simulink model "SPWM"  (R2018a)
settings: Solver=FixedStepDiscrete  StartTime=0.0  StopTime=Inf  FixedStep=1e-5  RelTol=1e-3  EnableMultiTasking=on
undefined symbols (not defined in the file or in its folder): Down, GPTRIP1SEL, GPTRIP2SEL, TZ1, TZ2, Up
libraries: idelinklib_common x48, c2837xDlib x27, c2802xlib x2, c2000lib x1, simulink x1
(part 1 of 2)
settings Model: ExtModeTrigDuration=8  Creator=ThinkPad  LastModifiedBy=ThinkPad
settings OptimizationCC: DefaultUnderspecifiedDataType=single  EnhancedBackFolding=on  PassReuseOutputArgsAs=Individual arguments  MaxStackSize=512  OptimizeBlockOrder=speed  DifferentSizesBufferReuse=on  OptimizationCustomize=off
settings DebuggingCC: ParameterTunabilityLossMsg=error
settings HardwareCC: ProdBitPerChar=16  ProdBitPerInt=16  ProdBitPerPointer=32  ProdBitPerSizeT=32  ProdBitPerPtrDiffT=32  ProdLargestAtomicInteger=Integer  ProdLargestAtomicFloat=None  ProdWordSize=16  ProdLongLongMode=on  ProdHWDeviceType=Texas Instruments->C2000
settings SFSimCC: MATLABDynamicMemAlloc=off
settings RTWCC: SystemTargetFile=ert.tlc  HardwareBoard=TI Delfino F2837xD  TLCOptions=-aInlineSetEventsForThisBaseRateFcn=TLC_FALSE -aSuppressMultiTaskScheduler=TLC_FALSE -aRateBasedStepFcn=1  TemplateMakefile=ert_default_tmf  GenerateReport=on  Toolchain=Texas Instruments Code Composer Studio (C2000)  IncludeHyperlinkInReport=on  LaunchReport=on  GenerateTraceInfo=on  GenerateTraceReport=on  GenerateTraceReportSl=on  GenerateTraceReportSf=on  GenerateTraceReportEml=on
settings RTWCC: CustomHeaderCode=|
  | nt i=0;
  | #define AD_ADDRESS1 (int16 * )0x0081F00
settings CodeAppCC: ForceParamTrailComments=on  IgnoreCustomStorageClasses=off  OperatorAnnotations=on  SimulinkDataObjDesc=on  SFDataObjDesc=on  InsertBlockDesc=on
settings ERTTargetCC: TargetLangStandard=C99 (ISO)  CodeReplacementLibrary=TI C28x  RootIOFormat=Structure reference  EnableSignedLeftShifts=off

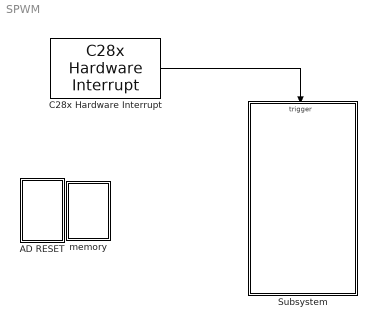
== system SPWM ==
  AD RESET : Subsystem
  C28x Hardware Interrupt : c2000lib/Scheduling/C28x Hardware Interrupt  irqnumbers=[3 1]  pienumbers=[1 2]  irqpriorities=[30 26]  irqpreempts=[0 0]  showinput=off  dspchiptype=C280X
      settings: SourceProductName=Embedded Coder Support Package for Texas Instruments C2000 Processors  SourceProductBaseCode=TIC2000
  Subsystem : Subsystem
  memory : Subsystem
  wires:
  C28x Hardware Interrupt/1 -> Subsystem/Trigger

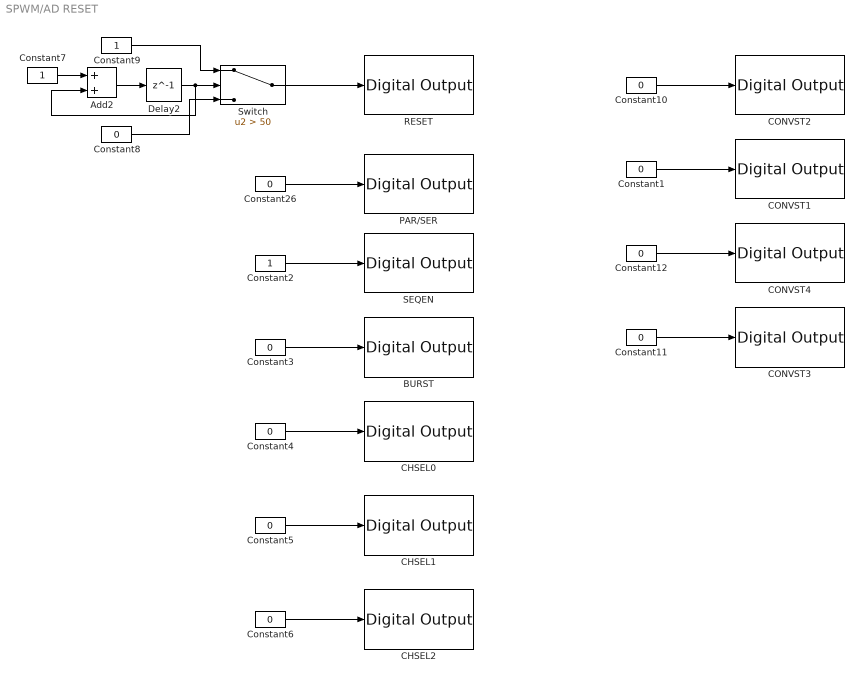
== system SPWM/AD RESET ==
  Add2 : Sum
  BURST : c2837xDlib/Digital Output  GPIO_Number=GPIO72~GPIO79  GPIO_Bit0=off  GPIO_BIT0_Toggle=off  GPIO_Bit1=off  GPIO_BIT1_Toggle=off  GPIO_Bit2=off  GPIO_BIT2_Toggle=off  GPIO_Bit3=off  GPIO_BIT3_Toggle=off  GPIO_Bit4=on  GPIO_BIT4_Toggle=off  GPIO_Bit5=off  GPIO_BIT5_Toggle=off  GPIO_Bit6=off  GPIO_BIT6_Toggle=off  GPIO_Bit7=off  GPIO_BIT7_Toggle=off
      settings: SourceProductName=Embedded Coder Support Package for Texas Instruments C2000 Processors  SourceProductBaseCode=TIC2000
  CHSEL0 : c2837xDlib/Digital Output  GPIO_Number=GPIO80~GPIO87  GPIO_Bit0=off  GPIO_BIT0_Toggle=off  GPIO_Bit1=off  GPIO_BIT1_Toggle=off  GPIO_Bit2=off  GPIO_BIT2_Toggle=off  GPIO_Bit3=on  GPIO_BIT3_Toggle=off  GPIO_Bit4=off  GPIO_BIT4_Toggle=off  GPIO_Bit5=off  GPIO_BIT5_Toggle=off  GPIO_Bit6=off  GPIO_BIT6_Toggle=off  GPIO_Bit7=off  GPIO_BIT7_Toggle=off
      settings: SourceProductName=Embedded Coder Support Package for Texas Instruments C2000 Processors  SourceProductBaseCode=TIC2000
  CHSEL1 : c2837xDlib/Digital Output  GPIO_Number=GPIO80~GPIO87  GPIO_Bit0=off  GPIO_BIT0_Toggle=off  GPIO_Bit1=on  GPIO_BIT1_Toggle=off  GPIO_Bit2=off  GPIO_BIT2_Toggle=off  GPIO_Bit3=off  GPIO_BIT3_Toggle=off  GPIO_Bit4=off  GPIO_BIT4_Toggle=off  GPIO_Bit5=off  GPIO_BIT5_Toggle=off  GPIO_Bit6=off  GPIO_BIT6_Toggle=off  GPIO_Bit7=off  GPIO_BIT7_Toggle=off
      settings: SourceProductName=Embedded Coder Support Package for Texas Instruments C2000 Processors  SourceProductBaseCode=TIC2000
  CHSEL2 : c2837xDlib/Digital Output  GPIO_Number=GPIO72~GPIO79  GPIO_Bit0=off  GPIO_BIT0_Toggle=off  GPIO_Bit1=off  GPIO_BIT1_Toggle=off  GPIO_Bit2=off  GPIO_BIT2_Toggle=off  GPIO_Bit3=off  GPIO_BIT3_Toggle=off  GPIO_Bit4=off  GPIO_BIT4_Toggle=off  GPIO_Bit5=off  GPIO_BIT5_Toggle=off  GPIO_Bit6=off  GPIO_BIT6_Toggle=off  GPIO_Bit7=on  GPIO_BIT7_Toggle=off
      settings: SourceProductName=Embedded Coder Support Package for Texas Instruments C2000 Processors  SourceProductBaseCode=TIC2000
  CONVST{1..4} (4 alike) : c2837xDlib/Digital Output  GPIO_Number=GPIO88~GPIO95  GPIO_Bit0=off  GPIO_BIT0_Toggle=off  GPIO_Bit1=on  GPIO_BIT1_Toggle=off  GPIO_Bit2=off  GPIO_BIT2_Toggle=off  GPIO_Bit3=off  GPIO_BIT3_Toggle=off  GPIO_Bit4=off  GPIO_BIT4_Toggle=off  GPIO_Bit5=off  GPIO_BIT5_Toggle=off  GPIO_Bit6=off  GPIO_BIT6_Toggle=off  GPIO_Bit7=off  GPIO_BIT7_Toggle=off
      settings: SourceProductName=Embedded Coder Support Package for Texas Instruments C2000 Processors  SourceProductBaseCode=TIC2000
  Constant{1,3..6,8,10..12,26} (10 alike) : Constant  Value=0  OutDataTypeStr=boolean
  Constant2 : Constant  OutDataTypeStr=boolean
  Constant7 : Constant  OutDataTypeStr=boolean
  Constant9 : Constant  OutDataTypeStr=boolean
  Delay2 : Delay  DelayLength=1
  PAR/SER : c2837xDlib/Digital Output  GPIO_Number=GPIO72~GPIO79  GPIO_Bit0=off  GPIO_BIT0_Toggle=off  GPIO_Bit1=off  GPIO_BIT1_Toggle=off  GPIO_Bit2=off  GPIO_BIT2_Toggle=off  GPIO_Bit3=off  GPIO_BIT3_Toggle=off  GPIO_Bit4=off  GPIO_BIT4_Toggle=off  GPIO_Bit5=off  GPIO_BIT5_Toggle=off  GPIO_Bit6=on  GPIO_BIT6_Toggle=off  GPIO_Bit7=off  GPIO_BIT7_Toggle=off
      settings: SourceProductName=Embedded Coder Support Package for Texas Instruments C2000 Processors  SourceProductBaseCode=TIC2000
  RESET : c2837xDlib/Digital Output  GPIO_Number=GPIO88~GPIO95  GPIO_Bit0=off  GPIO_BIT0_Toggle=off  GPIO_Bit1=off  GPIO_BIT1_Toggle=off  GPIO_Bit2=off  GPIO_BIT2_Toggle=off  GPIO_Bit3=off  GPIO_BIT3_Toggle=off  GPIO_Bit4=off  GPIO_BIT4_Toggle=off  GPIO_Bit5=on  GPIO_BIT5_Toggle=off  GPIO_Bit6=off  GPIO_BIT6_Toggle=off  GPIO_Bit7=off  GPIO_BIT7_Toggle=off
      settings: SourceProductName=Embedded Coder Support Package for Texas Instruments C2000 Processors  SourceProductBaseCode=TIC2000
  SEQEN : c2837xDlib/Digital Output  GPIO_Number=GPIO80~GPIO87  GPIO_Bit0=on  GPIO_BIT0_Toggle=off  GPIO_Bit1=off  GPIO_BIT1_Toggle=off  GPIO_Bit2=off  GPIO_BIT2_Toggle=off  GPIO_Bit3=off  GPIO_BIT3_Toggle=off  GPIO_Bit4=off  GPIO_BIT4_Toggle=off  GPIO_Bit5=off  GPIO_BIT5_Toggle=off  GPIO_Bit6=off  GPIO_BIT6_Toggle=off  GPIO_Bit7=off  GPIO_BIT7_Toggle=off
      settings: SourceProductName=Embedded Coder Support Package for Texas Instruments C2000 Processors  SourceProductBaseCode=TIC2000
  Switch : Switch  Criteria=u2 > Threshold  Threshold=50
  wires:
  Constant4/1 -> CHSEL0/1
  Delay2/1 -> Add2/2, Switch/2
  Constant5/1 -> CHSEL1/1
  Constant3/1 -> BURST/1
  Constant8/1 -> Switch/3
  Add2/1 -> Delay2/1
  Switch/1 -> RESET/1
  Constant7/1 -> Add2/1
  Constant6/1 -> CHSEL2/1
  Constant2/1 -> SEQEN/1
  Constant9/1 -> Switch/1
  Constant26/1 -> PAR/SER/1
  Constant10/1 -> CONVST2/1
  Constant1/1 -> CONVST1/1
  Constant11/1 -> CONVST3/1
  Constant12/1 -> CONVST4/1

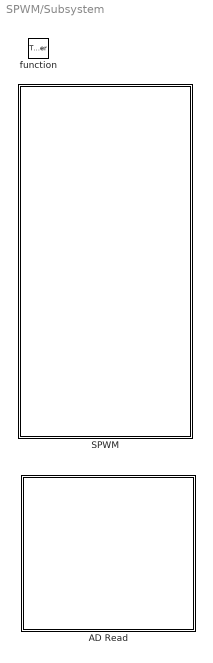
== system SPWM/Subsystem ==
  function : TriggerPort  TriggerType=function-call  VariantControl=(inherit)  SampleTime=1e-5
  AD Read : Subsystem
  SPWM : Subsystem

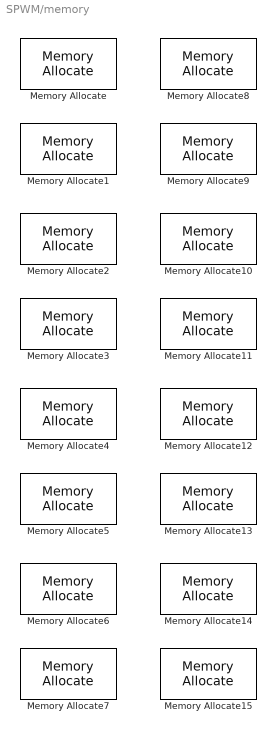
== system SPWM/memory ==
  Memory Allocate : idelinklib_common/Memory Allocate  variableName=V0A  alignThisVariable=off  memoryAlignmentBoundary=4  dataType=int16  specifyQualifier=off  typeQualifier=volatile  dataDimension=1  specifyMemorySection=off  memorySection=Sector A  bindMemorySection=on  sectionStartAddress=hex2dec('00080000')  initializeMemory=on  initialValue=0
  Memory Allocate1 : idelinklib_common/Memory Allocate  variableName=V0B  alignThisVariable=off  memoryAlignmentBoundary=4  dataType=int16  specifyQualifier=off  typeQualifier=volatile  dataDimension=1  specifyMemorySection=off  memorySection=Sector A  bindMemorySection=on  sectionStartAddress=hex2dec('00080000')  initializeMemory=on  initialValue=0
  Memory Allocate10 : idelinklib_common/Memory Allocate  variableName=V5A  alignThisVariable=off  memoryAlignmentBoundary=4  dataType=int16  specifyQualifier=off  typeQualifier=volatile  dataDimension=1  specifyMemorySection=off  memorySection=Sector A  bindMemorySection=on  sectionStartAddress=hex2dec('00080000')  initializeMemory=on  initialValue=0
  Memory Allocate11 : idelinklib_common/Memory Allocate  variableName=V5B  alignThisVariable=off  memoryAlignmentBoundary=4  dataType=int16  specifyQualifier=off  typeQualifier=volatile  dataDimension=1  specifyMemorySection=off  memorySection=Sector A  bindMemorySection=on  sectionStartAddress=hex2dec('00080000')  initializeMemory=on  initialValue=0
  Memory Allocate12 : idelinklib_common/Memory Allocate  variableName=V6A  alignThisVariable=off  memoryAlignmentBoundary=4  dataType=int16  specifyQualifier=off  typeQualifier=volatile  dataDimension=1  specifyMemorySection=off  memorySection=Sector A  bindMemorySection=on  sectionStartAddress=hex2dec('00080000')  initializeMemory=on  initialValue=0
  Memory Allocate13 : idelinklib_common/Memory Allocate  variableName=V6B  alignThisVariable=off  memoryAlignmentBoundary=4  dataType=int16  specifyQualifier=off  typeQualifier=volatile  dataDimension=1  specifyMemorySection=off  memorySection=Sector A  bindMemorySection=on  sectionStartAddress=hex2dec('00080000')  initializeMemory=on  initialValue=0
  Memory Allocate14 : idelinklib_common/Memory Allocate  variableName=V7A  alignThisVariable=off  memoryAlignmentBoundary=4  dataType=int16  specifyQualifier=off  typeQualifier=volatile  dataDimension=1  specifyMemorySection=off  memorySection=Sector A  bindMemorySection=on  sectionStartAddress=hex2dec('00080000')  initializeMemory=on  initialValue=0
  Memory Allocate15 : idelinklib_common/Memory Allocate  variableName=V7B  alignThisVariable=off  memoryAlignmentBoundary=4  dataType=int16  specifyQualifier=off  typeQualifier=volatile  dataDimension=1  specifyMemorySection=off  memorySection=Sector A  bindMemorySection=on  sectionStartAddress=hex2dec('00080000')  initializeMemory=on  initialValue=0
  Memory Allocate2 : idelinklib_common/Memory Allocate  variableName=V1A  alignThisVariable=off  memoryAlignmentBoundary=4  dataType=int16  specifyQualifier=off  typeQualifier=volatile  dataDimension=1  specifyMemorySection=off  memorySection=Sector A  bindMemorySection=on  sectionStartAddress=hex2dec('00080000')  initializeMemory=on  initialValue=0
  Memory Allocate3 : idelinklib_common/Memory Allocate  variableName=V1B  alignThisVariable=off  memoryAlignmentBoundary=4  dataType=int16  specifyQualifier=off  typeQualifier=volatile  dataDimension=1  specifyMemorySection=off  memorySection=Sector A  bindMemorySection=on  sectionStartAddress=hex2dec('00080000')  initializeMemory=on  initialValue=0
  Memory Allocate4 : idelinklib_common/Memory Allocate  variableName=V2A  alignThisVariable=off  memoryAlignmentBoundary=4  dataType=int16  specifyQualifier=off  typeQualifier=volatile  dataDimension=1  specifyMemorySection=off  memorySection=Sector A  bindMemorySection=on  sectionStartAddress=hex2dec('00080000')  initializeMemory=on  initialValue=0
  Memory Allocate5 : idelinklib_common/Memory Allocate  variableName=V2B  alignThisVariable=off  memoryAlignmentBoundary=4  dataType=int16  specifyQualifier=off  typeQualifier=volatile  dataDimension=1  specifyMemorySection=off  memorySection=Sector A  bindMemorySection=on  sectionStartAddress=hex2dec('00080000')  initializeMemory=on  initialValue=0
  Memory Allocate6 : idelinklib_common/Memory Allocate  variableName=V3A  alignThisVariable=off  memoryAlignmentBoundary=4  dataType=int16  specifyQualifier=off  typeQualifier=volatile  dataDimension=1  specifyMemorySection=off  memorySection=Sector A  bindMemorySection=on  sectionStartAddress=hex2dec('00080000')  initializeMemory=on  initialValue=0
  Memory Allocate7 : idelinklib_common/Memory Allocate  variableName=V3B  alignThisVariable=off  memoryAlignmentBoundary=4  dataType=int16  specifyQualifier=off  typeQualifier=volatile  dataDimension=1  specifyMemorySection=off  memorySection=Sector A  bindMemorySection=on  sectionStartAddress=hex2dec('00080000')  initializeMemory=on  initialValue=0
  Memory Allocate8 : idelinklib_common/Memory Allocate  variableName=V4A  alignThisVariable=off  memoryAlignmentBoundary=4  dataType=int16  specifyQualifier=off  typeQualifier=volatile  dataDimension=1  specifyMemorySection=off  memorySection=Sector A  bindMemorySection=on  sectionStartAddress=hex2dec('00080000')  initializeMemory=on  initialValue=0
  Memory Allocate9 : idelinklib_common/Memory Allocate  variableName=V4B  alignThisVariable=off  memoryAlignmentBoundary=4  dataType=int16  specifyQualifier=off  typeQualifier=volatile  dataDimension=1  specifyMemorySection=off  memorySection=Sector A  bindMemorySection=on  sectionStartAddress=hex2dec('00080000')  initializeMemory=on  initialValue=0

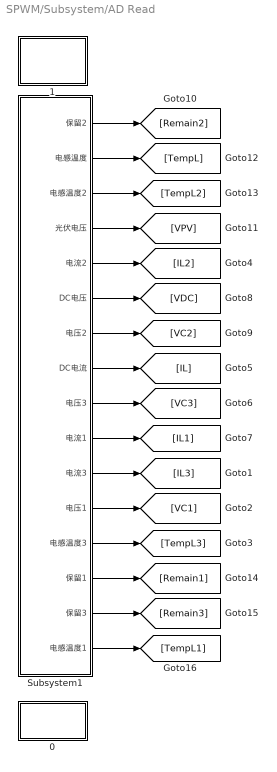
== system SPWM/Subsystem/AD Read ==
  0 : Subsystem
  1 : Subsystem
  Subsystem1 : Subsystem
  wires:
  Subsystem1/16(电感温度1) -> [TempL1]
  Subsystem1/15(保留3) -> [Remain3]
  Subsystem1/14(保留1) -> [Remain1]
  Subsystem1/13(电感温度3) -> [TempL3]
  Subsystem1/12(电压1) -> [VC1]
  Subsystem1/11(电流3) -> [IL3]
  Subsystem1/10(电流1) -> [IL1]
  Subsystem1/9(电压3) -> [VC3]
  Subsystem1/7(电压2) -> [VC2]
  Subsystem1/6(DC电压) -> [VDC]
  Subsystem1/5(电流2) -> [IL2]
  Subsystem1/3(电感温度2) -> [TempL2]
  Subsystem1/8(DC电流) -> [IL]
  Subsystem1/2(电感温度) -> [TempL]
  Subsystem1/4(光伏电压) -> [VPV]
  Subsystem1/1(保留2) -> [Remain2]

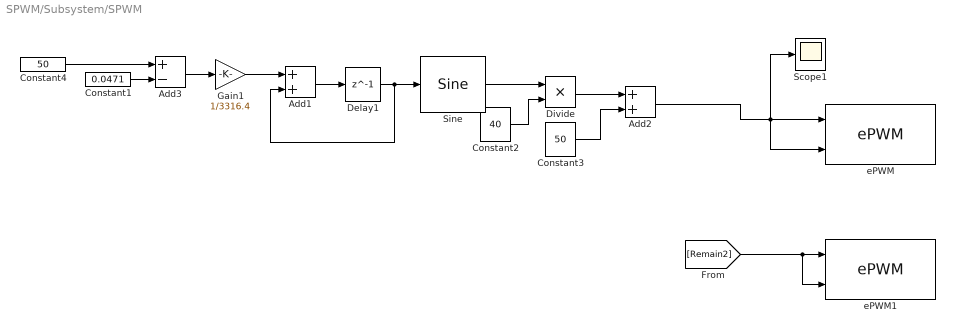
== system SPWM/Subsystem/SPWM ==
  Add1 : Sum
  Add2 : Sum
  Add3 : Sum  Inputs=+-
  Constant1 : Constant  Value=0.0471  VectorParams1D=off
  Constant2 : Constant  Value=40  VectorParams1D=off
  Constant3 : Constant  Value=50  VectorParams1D=off
  Constant4 : Constant  Value=50  VectorParams1D=off
  Delay1 : Delay  DelayLength=1
  Divide : Product  Inputs=**
  Gain1 : Gain  Gain=1/3316.4
  Scope1 : Scope
  Sine : simulink/Lookup Tables/Sine  Formula=sin(2*pi*u)  NumDataPoints=(2^5)+1  OutputWordLength=16  InternalRulePriority=Precision
      settings: SourceProductName=Simulink
  ePWM : c2802xlib/ePWM  useModule=ePWM1  ePWMxLINKTBPRD=Not Linked  periodUnits=Clock cycles  timerSource=Specify via dialog  timerPeriod_clk=15000  timerPeriod_sec=0.0001  tbshadow=Counter equals to zero  countingMode=Up-Down  phaseActiveEnable=Disable  phaseDirection=Count down after sync  phaseActive=0  synchronizationEnable=off  dcaevt1Sync=off  dcbevt1Sync=off  synchronizationOption=Disable  clockPrescale=1  HSclockPrescale=1  enswap=off  ePWMxAStatus=on  ePWMxAactionLogic1=Set  ePWMxAactionLogic2=Clear  ePWMxAactionLogic3=Clear  ePWMxAactionLogic4=Set  ePWMxAactionLogic5=Do nothing  ePWMxAactionLogic6=Do nothing  ePWMxALoadMode=Load on counter equals to zero (CTR=Zero)  ePWMxACSFenable=off  ePWMxACSFvalue=Forcing disable  ePWMxASFreload=Zero  ePWMxBStatus=on  ePWMxBactionLogic1=Set  ePWMxBactionLogic2=Clear  ePWMxBactionLogic3=Do nothing  ePWMxBactionLogic4=Do nothing  ePWMxBactionLogic5=Clear  ePWMxBactionLogic6=Set  ePWMxBLoadMode=Load on counter equals to zero (CTR=Zero)  ePWMxBCSFenable=off  ePWMxBCSFvalue=Forcing disable  ePWMxBSFreload=Zero  ePWNxBOutWay=on  ePWMxLINKCMPA=Not Linked  CMPAUnits=Percentages  CMPASource=Input port  CMPAValue_per=0  CMPAValue_clk=0  enCMPAshadow=Counter equals to zero  ePWMxLINKCMPB=Not Linked  CMPBUnits=Percentages  CMPBSource=Input port  CMPBValue_per=0  CMPBValue_clk=0  enCMPBshadow=Counter equals to zero  ePWMxLINKCMPC=Not Linked  CMPCUnits=Clock cycles  CMPCSource=Specify via dialog  CMPCValue_per=50  CMPCValue_clk=32000  enCMPCshadow=Counter equals to zero  ePWMxLINKCMPD=Not Linked  CMPDUnits=Clock cycles  CMPDSource=Specify via dialog  CMPDValue_per=50  CMPDValue_clk=32000  enCMPDshadow=Counter equals to zero  enableDBePWMxA=on  enableDBePWMxB=on  enhalfcycle=off  DBpolarity=Active high (AH)  DBedgeDelay=Positive  DBSource_ePWMxA=ePWMxA  DBSource_ePWMxB=ePWMxA  DBperiodSource=Specify via dialog  REDperiod=500  FEDperiod=500  adcstartModuleA=off  adcrequestEventA=First event  adcstartEventA=Digital Compare Module A Event 1 start of conversion (DCAEVT1.soc)  adcstartEventA_type2=Digital Compare Module A Event 1 start of conversion (DCAEVT1.soc)  adcstartModuleB=off  adcrequestEventB=First event  adcstartEventB=Counter equals to zero (CTR=Zero)  adcstartEventB_type2=Counter equals to zero (CTR=Zero)  intEn=on  intPrd=First event  intSel=Counter equals to zero (CTR=Zero)  intSel_type2=Counter equals to zero (CTR=Zero)  hrpe=off  enHRPWM=off  HRPWM_LoadMode=Counter equals to period (CTR=PRD)  HRPWM_CTLMode=Duty or Period control mode  HRPWM_EDGMode=Both edge  hrpeb=off  enHRPWMB=off  HRPWM_LoadModeB=Counter equals to zero (CTR=ZERO)  HRPWM_CTLModeB=Duty or Period control mode  HRPWM_EDGModeB=Both edge  enSFO=on  enautoconv=on  chopperEnable=off  chopperFrequency=1  chopperFirstwidth=1  chopperDuty=12.5%  tripZonesource=Specify via dialog  tzselOSHT1=off  tzselOSHT2=off  tzselOSHT3=off  tzselOSHDCAEV1=off  tzselOSHDCBEV1=off  tzselCBC1=off  tzselCBC2=off  tzselCBC3=off  tzselCBCDCAEV2=off  tzselCBCDCBEV2=off  tzselOSHT4=off  tzselOSHT5=off  tzselOSHT6=off  tzselCBC4=off  tzselCBC5=off  tzselCBC6=off  enTzOstIntr=off  enTzCbcIntr=off  enTzDCAEVT1Intr=off  enTzDCAEVT2Intr=off  enTzDCBEVT1Intr=off  enTzDCBEVT2Intr=off  ePWMxAforced=No action  ePWMxBforced=No action  DCAEVT1forced=No action  DCBEVT1forced=No action  DCAEVT2forced=No action  DCBEVT2forced=No action  dcah=Trip Zone 1 input (TZ1)  dcal=Trip Zone 2 input (TZ2)  dcbh=Trip Zone 1 input (TZ1)  dcbl=Trip Zone 2 input (TZ2)  dcah_type2=GPTRIP1SEL/(TZ1)  dcal_type2=GPTRIP2SEL/(TZ2)  dcbh_type2=GPTRIP1SEL/(TZ1)  dcbl_type2=GPTRIP2SEL/(TZ2)  gendcaevt1=Event disabled  gendcaevt2=Event disabled  gendcbevt1=Event disabled  gendcbevt2=Event disabled  dcaevt1src=DCAEVT1 with sync  dcaevt2src=DCAEVT2 with sync  dcbevt1src=DCBEVT1 with sync  dcbevt2src=DCBEVT2 with sync  pulsesel=Counter equals to zero (CTR=Zero)  blankinv=off  blankoffset=0  blankwidth=0  evsrcsel=Filtered version of DCAEVT1 (DCAEVT1FILT)  encape=off  PwmType=C2000_Type4
      settings: SourceProductName=Embedded Coder Support Package for Texas Instruments C2000 Processors
  ePWM1 : c2802xlib/ePWM  useModule=ePWM2  ePWMxLINKTBPRD=Not Linked  periodUnits=Clock cycles  timerSource=Specify via dialog  timerPeriod_clk=15000  timerPeriod_sec=0.0001  tbshadow=Counter equals to zero  countingMode=Up-Down  phaseActiveEnable=Disable  phaseDirection=Count down after sync  phaseActive=0  synchronizationEnable=off  dcaevt1Sync=off  dcbevt1Sync=off  synchronizationOption=Disable  clockPrescale=1  HSclockPrescale=1  enswap=off  ePWMxAStatus=on  ePWMxAactionLogic1=Set  ePWMxAactionLogic2=Clear  ePWMxAactionLogic3=Clear  ePWMxAactionLogic4=Set  ePWMxAactionLogic5=Do nothing  ePWMxAactionLogic6=Do nothing  ePWMxALoadMode=Load on counter equals to zero (CTR=Zero)  ePWMxACSFenable=off  ePWMxACSFvalue=Forcing disable  ePWMxASFreload=Zero  ePWMxBStatus=on  ePWMxBactionLogic1=Set  ePWMxBactionLogic2=Clear  ePWMxBactionLogic3=Do nothing  ePWMxBactionLogic4=Do nothing  ePWMxBactionLogic5=Clear  ePWMxBactionLogic6=Set  ePWMxBLoadMode=Load on counter equals to zero (CTR=Zero)  ePWMxBCSFenable=off  ePWMxBCSFvalue=Forcing disable  ePWMxBSFreload=Zero  ePWNxBOutWay=on  ePWMxLINKCMPA=Not Linked  CMPAUnits=Percentages  CMPASource=Input port  CMPAValue_per=0  CMPAValue_clk=0  enCMPAshadow=Counter equals to zero  ePWMxLINKCMPB=Not Linked  CMPBUnits=Percentages  CMPBSource=Input port  CMPBValue_per=0  CMPBValue_clk=0  enCMPBshadow=Counter equals to zero  ePWMxLINKCMPC=Not Linked  CMPCUnits=Clock cycles  CMPCSource=Specify via dialog  CMPCValue_per=50  CMPCValue_clk=32000  enCMPCshadow=Counter equals to zero  ePWMxLINKCMPD=Not Linked  CMPDUnits=Clock cycles  CMPDSource=Specify via dialog  CMPDValue_per=50  CMPDValue_clk=32000  enCMPDshadow=Counter equals to zero  enableDBePWMxA=on  enableDBePWMxB=on  enhalfcycle=off  DBpolarity=Active high (AH)  DBedgeDelay=Positive  DBSource_ePWMxA=ePWMxA  DBSource_ePWMxB=ePWMxA  DBperiodSource=Specify via dialog  REDperiod=500  FEDperiod=500  adcstartModuleA=off  adcrequestEventA=First event  adcstartEventA=Digital Compare Module A Event 1 start of conversion (DCAEVT1.soc)  adcstartEventA_type2=Digital Compare Module A Event 1 start of conversion (DCAEVT1.soc)  adcstartModuleB=off  adcrequestEventB=First event  adcstartEventB=Counter equals to zero (CTR=Zero)  adcstartEventB_type2=Counter equals to zero (CTR=Zero)  intEn=on  intPrd=First event  intSel=Counter equals to zero (CTR=Zero)  intSel_type2=Counter equals to zero (CTR=Zero)  hrpe=off  enHRPWM=off  HRPWM_LoadMode=Counter equals to period (CTR=PRD)  HRPWM_CTLMode=Duty or Period control mode  HRPWM_EDGMode=Both edge  hrpeb=off  enHRPWMB=off  HRPWM_LoadModeB=Counter equals to zero (CTR=ZERO)  HRPWM_CTLModeB=Duty or Period control mode  HRPWM_EDGModeB=Both edge  enSFO=on  enautoconv=on  chopperEnable=off  chopperFrequency=1  chopperFirstwidth=1  chopperDuty=12.5%  tripZonesource=Specify via dialog  tzselOSHT1=off  tzselOSHT2=off  tzselOSHT3=off  tzselOSHDCAEV1=off  tzselOSHDCBEV1=off  tzselCBC1=off  tzselCBC2=off  tzselCBC3=off  tzselCBCDCAEV2=off  tzselCBCDCBEV2=off  tzselOSHT4=off  tzselOSHT5=off  tzselOSHT6=off  tzselCBC4=off  tzselCBC5=off  tzselCBC6=off  enTzOstIntr=off  enTzCbcIntr=off  enTzDCAEVT1Intr=off  enTzDCAEVT2Intr=off  enTzDCBEVT1Intr=off  enTzDCBEVT2Intr=off  ePWMxAforced=No action  ePWMxBforced=No action  DCAEVT1forced=No action  DCBEVT1forced=No action  DCAEVT2forced=No action  DCBEVT2forced=No action  dcah=Trip Zone 1 input (TZ1)  dcal=Trip Zone 2 input (TZ2)  dcbh=Trip Zone 1 input (TZ1)  dcbl=Trip Zone 2 input (TZ2)  dcah_type2=GPTRIP1SEL/(TZ1)  dcal_type2=GPTRIP2SEL/(TZ2)  dcbh_type2=GPTRIP1SEL/(TZ1)  dcbl_type2=GPTRIP2SEL/(TZ2)  gendcaevt1=Event disabled  gendcaevt2=Event disabled  gendcbevt1=Event disabled  gendcbevt2=Event disabled  dcaevt1src=DCAEVT1 with sync  dcaevt2src=DCAEVT2 with sync  dcbevt1src=DCBEVT1 with sync  dcbevt2src=DCBEVT2 with sync  pulsesel=Counter equals to zero (CTR=Zero)  blankinv=off  blankoffset=0  blankwidth=0  evsrcsel=Filtered version of DCAEVT1 (DCAEVT1FILT)  encape=off  PwmType=C2000_Type4
      settings: SourceProductName=Embedded Coder Support Package for Texas Instruments C2000 Processors
  wires:
  Add2/1 -> ePWM/2, ePWM/1, Scope1/1
  [Remain2] -> ePWM1/2, ePWM1/1
  Sine/1 -> Divide/1
  Divide/1 -> Add2/1
  Add3/1 -> Gain1/1
  Constant1/1 -> Add3/2
  Constant3/1 -> Add2/2
  Constant4/1 -> Add3/1
  Delay1/1 -> Sine/1, Add1/2
  Constant2/1 -> Divide/2
  Gain1/1 -> Add1/1
  Add1/1 -> Delay1/1

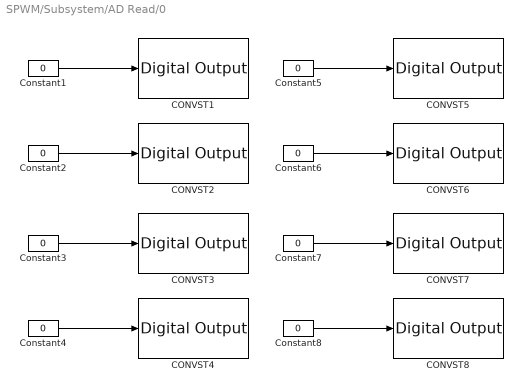
== system SPWM/Subsystem/AD Read/0 ==
  CONVST{1..8} (8 alike) : c2837xDlib/Digital Output  GPIO_Number=GPIO88~GPIO95  GPIO_Bit0=off  GPIO_BIT0_Toggle=off  GPIO_Bit1=on  GPIO_BIT1_Toggle=off  GPIO_Bit2=off  GPIO_BIT2_Toggle=off  GPIO_Bit3=off  GPIO_BIT3_Toggle=off  GPIO_Bit4=off  GPIO_BIT4_Toggle=off  GPIO_Bit5=off  GPIO_BIT5_Toggle=off  GPIO_Bit6=off  GPIO_BIT6_Toggle=off  GPIO_Bit7=off  GPIO_BIT7_Toggle=off
      settings: SourceProductName=Embedded Coder Support Package for Texas Instruments C2000 Processors  SourceProductBaseCode=TIC2000
  Constant{1..8} (8 alike) : Constant  Value=0  OutDataTypeStr=boolean
  wires:
  Constant1/1 -> CONVST1/1
  Constant2/1 -> CONVST2/1
  Constant4/1 -> CONVST4/1
  Constant3/1 -> CONVST3/1
  Constant7/1 -> CONVST7/1
  Constant8/1 -> CONVST8/1
  Constant6/1 -> CONVST6/1
  Constant5/1 -> CONVST5/1

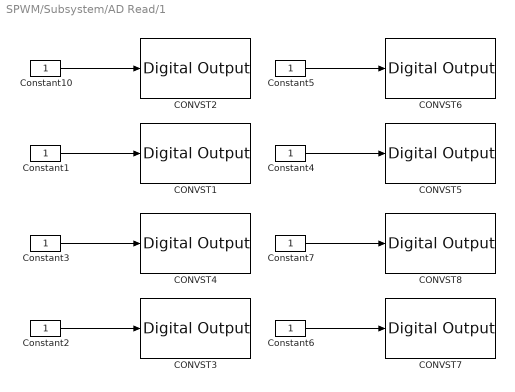
== system SPWM/Subsystem/AD Read/1 ==
  CONVST{1..8} (8 alike) : c2837xDlib/Digital Output  GPIO_Number=GPIO88~GPIO95  GPIO_Bit0=off  GPIO_BIT0_Toggle=off  GPIO_Bit1=on  GPIO_BIT1_Toggle=off  GPIO_Bit2=off  GPIO_BIT2_Toggle=off  GPIO_Bit3=off  GPIO_BIT3_Toggle=off  GPIO_Bit4=off  GPIO_BIT4_Toggle=off  GPIO_Bit5=off  GPIO_BIT5_Toggle=off  GPIO_Bit6=off  GPIO_BIT6_Toggle=off  GPIO_Bit7=off  GPIO_BIT7_Toggle=off
      settings: SourceProductName=Embedded Coder Support Package for Texas Instruments C2000 Processors  SourceProductBaseCode=TIC2000
  Constant{1..7,10} (8 alike) : Constant  OutDataTypeStr=boolean
  wires:
  Constant10/1 -> CONVST2/1
  Constant1/1 -> CONVST1/1
  Constant2/1 -> CONVST3/1
  Constant3/1 -> CONVST4/1
  Constant7/1 -> CONVST8/1
  Constant6/1 -> CONVST7/1
  Constant4/1 -> CONVST5/1
  Constant5/1 -> CONVST6/1
